simulink model "model_wahadlo"  (R2022b)
settings: Solver=ode4  StartTime=0.0  StopTime=100  FixedStep=0.01  RelTol=1e-3
settings Model: Creator=bm50345  LastModifiedBy=bm50345

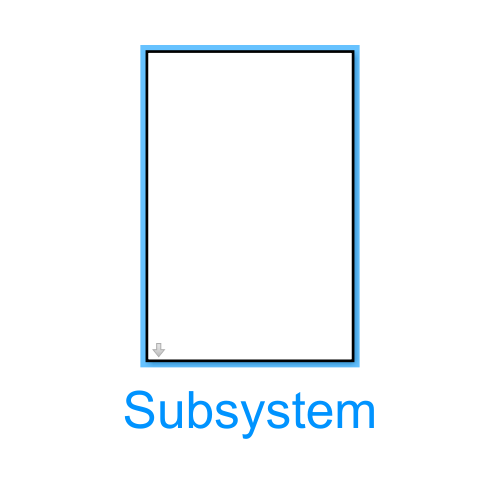
[thumbnail: Simulink's stored preview of the top-level diagram]
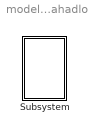
== system model_wahadlo ==
  Subsystem : Subsystem  mask{m=10, l=3, k=1, g=10, fi1=0, fi0=90}
      mask prompts: m "masa"; l "dlugosc"; k "tlumienie"; g "grawitacja"; fi1 "predkosc"; fi0 "kat"

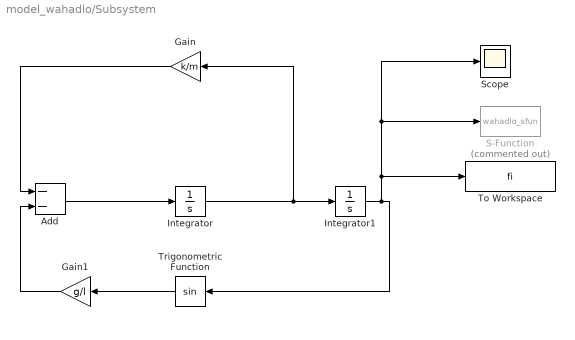
== system model_wahadlo/Subsystem ==
  Add : Sum  Inputs=--
  Gain : Gain  Gain=k/m
  Gain1 : Gain  Gain=g/l
  Integrator : Integrator  InitialCondition=fi1 * pi / 180
  Integrator1 : Integrator  InitialCondition=fi0 * pi / 180
  S-Function : S-Function  Commented=on  FunctionName=wahadlo_sfun  Parameters=l,m,fi0  SFunctionDeploymentMode=off  EnableBusSupport=off
  Scope : Scope
  To Workspace : ToWorkspace  VariableName=fi  SampleTime=-1
  Trigonometric Function : Trigonometry
  wires:
  Gain/1 -> Add/1
  Integrator1/1 -> To Workspace/1, S-Function/1, Scope/1, Trigonometric Function/1
  Integrator/1 -> Gain/1, Integrator1/1
  Add/1 -> Integrator/1
  Trigonometric Function/1 -> Gain1/1
  Gain1/1 -> Add/2
